simulink model "practica_10"  (Simulink 5.0)
settings: Solver=ode45  StartTime=0.0  StopTime=100.0  FixedStep=.1  MaxStep=.1*ts  RelTol=1e-4
undefined symbols (not defined in the file): ts
settings Model: ExtModeTrigMode=oneshot  ExtModeArmWhenConnect=off  LimitDataPoints=off  BlockReductionOpt=off  BooleanDataType=off

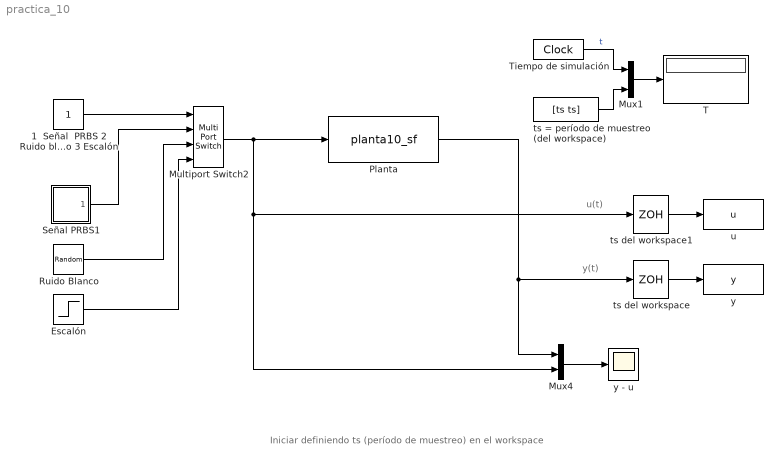
== system practica_10 ==
  note: y(t)
  note: u(t)
  note: Iniciar definiendo ts (período de muestreo) en el workspace
  1  Señal  PRBS 2 Ruido blanco 3 Escalón : Constant
  Escalón : Step  Time=0  SampleTime=0
  Multiport Switch2 : MultiPortSwitch  Inputs=3  SaturateOnIntegerOverflow=on  InputSameDT=on
  Mux1 : Mux  Inputs=2
  Mux4 : Mux  Inputs=2
  Planta : S-Function  FunctionName=planta10_sf  SFunctionModules=""  mask{rtw_sf_name=planta10_sf, showVar=off}
      mask prompts: rtw_sf_name "Generated S-function name (model_sf):"; showVar "Show module list"
      mask help: Real-Time Workshop generated S-function.
      mask init:
      | displist = '';
      | if ~strcmp(get_param(gcb, 'FunctionName'), rtw_sf_name);
      |   set_param(gcb, 'FunctionName', rtw_sf_name);
      | end
      | if  showVar & exist('rtwsfunc') == 2
      |   tmplist = rtwsfunc(rtw_sf_name,gcb);
      |   tmplist = ['\nList of Modules:\n', tmplist];
      | elseif showVar
      |   tmplist = '\nList of Modules:\nRTW not licensed\n';
      | end
      | if showVar
      |   displist = tmplist;
      | end
      settings: CopyFcn=set_param(gcb,'linkstatus','none')
      mask Help: web(['file://',docroot,'/toolbox/rtw/rtwsfcn.html']);
      mask Display:
      | port_label('input',1,'u(t)');
      | port_label('output',1,'y(t)');
  Ruido Blanco : RandomNumber  SampleTime=0
  Señal PRBS1 : Subsystem
  T : Display
  Tiempo de simulación : DigitalClock  SampleTime=.1
  ts = período de muestreo (del workspace) : FromWorkspace  VariableName=[ts ts]  SampleTime=0
  ts del workspace : ZeroOrderHold  SampleTime=ts
  ts del workspace1 : ZeroOrderHold  SampleTime=ts
  u : ToWorkspace  VariableName=u  SampleTime=ts  SaveFormat=Array
  y : ToWorkspace  VariableName=y  SampleTime=ts  SaveFormat=Array
  y - u : Scope
  wires:
  1  Señal  PRBS 2 Ruido blanco 3 Escalón/1 -> Multiport Switch2/1
  Ruido Blanco/1 -> Multiport Switch2/3
  Mux4/1 -> y - u/1
  Planta/1 -> ts del workspace/1, Mux4/1
  Multiport Switch2/1 -> Mux4/2, ts del workspace1/1, Planta/1
  Escalón/1 -> Multiport Switch2/4
  Señal PRBS1/1(u ( t )) -> Multiport Switch2/2
  ts del workspace/1 -> y/1
  ts = período de muestreo (del workspace)/1 -> Mux1/2
  Tiempo de simulación/1 -> Mux1/1  "t"
  Mux1/1 -> T/1
  ts del workspace1/1 -> u/1

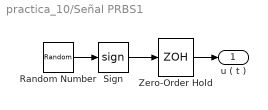
== system practica_10/Señal PRBS1 ==
  Random Number : RandomNumber  SampleTime=0
  Sign : Signum
  Zero-Order Hold : ZeroOrderHold  SampleTime=ts
  u ( t ) : Outport
  wires:
  Zero-Order Hold/1 -> u ( t )/1
  Sign/1 -> Zero-Order Hold/1
  Random Number/1 -> Sign/1
